simulink model "Scenario_17_v2"  (R2020b)
settings: Solver=ode1  StartTime=0.0  StopTime=10  FixedStep=Ts  MaxStep=Ts  MinStep=Ts/50  RelTol=1e-3
values from neighbouring files (symbols this model uses):
  c0 = c0_zeb    (= 6.57988e-09)    [Scenario_17_parameters_v2.m]    (also in Scenario_1_parameters_v2.m; Scenario_2_parameters_v2.m; Scenario_3_parameters_v2.m)
  c1 = c1_zeb    (= 9.15905e-09)    [Scenario_17_parameters_v2.m]    (also in Scenario_1_parameters_v2.m; Scenario_2_parameters_v2.m; Scenario_3_parameters_v2.m)
  fg = 50    [Scenario_17_parameters_v2.m]    (also in Scenario_1_parameters_v2.m; Scenario_2_parameters_v2.m; Scenario_3_parameters_v2.m)
  G11gen = 0.50    (= 0.5)    [Scenario_17_parameters_v2.m]
  G1gen = 0.4692    [Scenario_17_parameters_v2.m]    (also in Scenario_1_parameters_v2.m = 0.1; Scenario_2_parameters_v2.m = 0.298581; Scenario_3_parameters_v2.m = 0.65)
  G5gen = 0.75    [Scenario_17_parameters_v2.m]    (also in Scenario_1_parameters_v2.m = 0.8; Scenario_2_parameters_v2.m = 0.8; Scenario_3_parameters_v2.m = 0.705)
  G6gen = 0.90    (= 0.9)    [Scenario_17_parameters_v2.m]    (also in Scenario_1_parameters_v2.m; Scenario_2_parameters_v2.m = 0.81797; Scenario_3_parameters_v2.m = 0.45)
  G7gen = 0.20    (= 0.2)    [Scenario_17_parameters_v2.m]    (also in Scenario_1_parameters_v2.m = 0.5227; Scenario_2_parameters_v2.m = 0.5098; Scenario_3_parameters_v2.m = 0.4)
  G8gen = 0.58    [Scenario_17_parameters_v2.m]    (also in Scenario_3_parameters_v2.m = 0.65)
  G9gen = 0.8833    [Scenario_17_parameters_v2.m]    (also in Scenario_3_parameters_v2.m = 0.9)
  Iovc = 1.2    [Scenario_17_parameters_v2.m]    (also in Scenario_1_parameters_v2.m; Scenario_2_parameters_v2.m; Scenario_3_parameters_v2.m)
  l0 = l0_zeb    (= 0.00368)    [Scenario_17_parameters_v2.m]    (also in Scenario_1_parameters_v2.m; Scenario_2_parameters_v2.m; Scenario_3_parameters_v2.m)
  l1 = l1_zeb    (= 0.00128)    [Scenario_17_parameters_v2.m]    (also in Scenario_1_parameters_v2.m; Scenario_2_parameters_v2.m; Scenario_3_parameters_v2.m)
  L11dem = 0.02    [Scenario_17_parameters_v2.m]
  L12dem = 0.01    [Scenario_17_parameters_v2.m]    (also in Scenario_3_parameters_v2.m = 0.02)
  L1dem = 0.25    [Scenario_17_parameters_v2.m]    (also in Scenario_3_parameters_v2.m = 0.1)
  L3dem = 0.30    (= 0.3)    [Scenario_17_parameters_v2.m]    (also in Scenario_1_parameters_v2.m = 0.1; Scenario_2_parameters_v2.m = 0.1; Scenario_3_parameters_v2.m = 0.2)
  L5dem = 0.25    [Scenario_17_parameters_v2.m]    (also in Scenario_1_parameters_v2.m = 0.35; Scenario_2_parameters_v2.m = 0.35; Scenario_3_parameters_v2.m = 0.1)
  L9dem = 0.15    [Scenario_17_parameters_v2.m]    (also in Scenario_3_parameters_v2.m = 0.1)
  Pr = Sr*PF    (= 1600500000)    [Scenario_17_parameters_v2.m]    (also in Scenario_1_parameters_v2.m = 1472500000; Scenario_2_parameters_v2.m = 1805000000; Scenario_3_parameters_v2.m = 12740000000)
  Qr = sqrt(Sr^2 - Pr^2)    [Scenario_17_parameters_v2.m]    (also in Scenario_1_parameters_v2.m; Scenario_2_parameters_v2.m; Scenario_3_parameters_v2.m)
  r0 = r0_zeb    (= 0.39362)    [Scenario_17_parameters_v2.m]    (also in Scenario_1_parameters_v2.m; Scenario_2_parameters_v2.m; Scenario_3_parameters_v2.m)
  r1 = r1_zeb    (= 0.06862)    [Scenario_17_parameters_v2.m]    (also in Scenario_1_parameters_v2.m; Scenario_2_parameters_v2.m; Scenario_3_parameters_v2.m)
  Rtpu = Xtpu/40    (= 0.0025)    [Scenario_17_parameters_v2.m]    (also in Scenario_1_parameters_v2.m = 0.00375; Scenario_2_parameters_v2.m = 0.00375; Scenario_3_parameters_v2.m)
  S11non = 50e6    (= 50000000)    [Scenario_17_parameters_v2.m]
  S1non = 700e6    (= 700000000)    [Scenario_17_parameters_v2.m]    (also in Scenario_1_parameters_v2.m = 400000000; Scenario_2_parameters_v2.m = 400000000; Scenario_3_parameters_v2.m = 1000000000)
  S5non = 400e6    (= 400000000)    [Scenario_17_parameters_v2.m]    (also in Scenario_1_parameters_v2.m = 500000000; Scenario_2_parameters_v2.m = 500000000; Scenario_3_parameters_v2.m = 2000000000)
  S6non = 150e6    (= 150000000)    [Scenario_17_parameters_v2.m]    (also in Scenario_1_parameters_v2.m = 400000000; Scenario_2_parameters_v2.m = 400000000; Scenario_3_parameters_v2.m = 3000000000)
  S7non = 1500e6    (= 1500000000)    [Scenario_17_parameters_v2.m]    (also in Scenario_1_parameters_v2.m = 200000000; Scenario_2_parameters_v2.m = 200000000; Scenario_3_parameters_v2.m = 4000000000)
  S8non = 600e6    (= 600000000)    [Scenario_17_parameters_v2.m]    (also in Scenario_3_parameters_v2.m = 2000000000)
  S9non = 200e6    (= 200000000)    [Scenario_17_parameters_v2.m]    (also in Scenario_3_parameters_v2.m = 1500000000)
  tonvsc = 0    [Scenario_17_parameters_v2.m]    (also in Scenario_1_parameters_v2.m; Scenario_2_parameters_v2.m; Scenario_3_parameters_v2.m = 0.0001)
  Ts = 50e-6    (= 5e-05)    [Scenario_17_parameters_v2.m]    (also in Scenario_1_parameters_v2.m = 0.0002; Scenario_2_parameters_v2.m = 2e-05; Scenario_3_parameters_v2.m = 0.0001)
  Vhv = 220e3    (= 220000)    [Scenario_17_parameters_v2.m]    (also in Scenario_1_parameters_v2.m; Scenario_2_parameters_v2.m; Scenario_3_parameters_v2.m)
  Vmv = 22e3    (= 22000)    [Scenario_17_parameters_v2.m]    (also in Scenario_1_parameters_v2.m; Scenario_2_parameters_v2.m; Scenario_3_parameters_v2.m)
  w_pll = 2*pi*80    (= 502.654824574)    [Scenario_17_parameters_v2.m]    (also in Scenario_1_parameters_v2.m; Scenario_2_parameters_v2.m; Scenario_3_parameters_v2.m)
  wc1 = wsw1/10    (= 848.230016469)    [Scenario_17_parameters_v2.m]    (also in Scenario_1_parameters_v2.m; Scenario_2_parameters_v2.m; Scenario_3_parameters_v2.m)
  wdc1 = wc1/10    (= 84.8230016469)    [Scenario_17_parameters_v2.m]    (also in Scenario_1_parameters_v2.m; Scenario_2_parameters_v2.m; Scenario_3_parameters_v2.m)
  wpq1 = wc1/10    (= 84.8230016469)    [Scenario_17_parameters_v2.m]    (also in Scenario_1_parameters_v2.m; Scenario_2_parameters_v2.m; Scenario_3_parameters_v2.m)
  wsw1 = ksw1*2*pi*fg    (= 8482.30016469)    [Scenario_17_parameters_v2.m]    (also in Scenario_1_parameters_v2.m; Scenario_2_parameters_v2.m; Scenario_3_parameters_v2.m)
  Xtpu = 0.10    (= 0.1)    [Scenario_17_parameters_v2.m]    (also in Scenario_1_parameters_v2.m = 0.15; Scenario_2_parameters_v2.m = 0.15; Scenario_3_parameters_v2.m)
undefined symbols (not defined in the file or in its folder): D11, Delta, Newton, Raphson
libraries: powerlib x349, simulink_extras x215, powerlib_meascontrol x165, pid_lib x81, simulink x48, eeTransforms x42, spsFirstOrderFilterLib x28, eePwmGeneratorTwoLevel x7
(part 2 of 31)

== system Scenario_17_v2/B7 ==
  Current Measurement : powerlib/Measurements/Current Measurement  PhasorSimulation=off  OutputType=Complex  PSBequivalent=0
  Current Measurement1 : powerlib/Measurements/Current Measurement  PhasorSimulation=off  OutputType=Complex  PSBequivalent=0
  Current Measurement2 : powerlib/Measurements/Current Measurement  PhasorSimulation=off  OutputType=Complex  PSBequivalent=0
  Gain : Gain
  Gain1 : Gain
  Ground : powerlib/Elements/Ground  LConnTagsString=a
  Ground1 : powerlib/Elements/Ground  LConnTagsString=a
  Ground2 : powerlib/Elements/Ground  LConnTagsString=a
  Load Flow Bus : powerlib/Measurements/Load Flow Bus  LConnTagsString=a  Phases=single  Connectors=on one side  ID=BUS7  Vbase=Vhv  Vref=1  Vangle=0  VLF=1  VLFb=1  VLFc=1  angleLF=0  angleLFb=0  angleLFc=0
  Mux : Mux  Inputs=3
  Mux1 : Mux  Inputs=3
  Voltage Measurement : powerlib/Measurements/Voltage Measurement  PhasorSimulation=off  OutputType=Complex  PSBequivalent=0
  Voltage Measurement1 : powerlib/Measurements/Voltage Measurement  PhasorSimulation=off  OutputType=Complex  PSBequivalent=0
  Voltage Measurement2 : powerlib/Measurements/Voltage Measurement  PhasorSimulation=off  OutputType=Complex  PSBequivalent=0
  A : PMIOPort  Side=Left
  B : PMIOPort  Port=2  Side=Left
  C : PMIOPort  Port=3  Side=Left
  a : PMIOPort  Port=4  Side=Right
  b : PMIOPort  Port=5  Side=Right
  c : PMIOPort  Port=6  Side=Right
  tag scope: I7=global, V7=global
  wires:
  Voltage Measurement2/1 -> Mux/3
  Voltage Measurement1/1 -> Mux/2
  Voltage Measurement/1 -> Mux/1
  Current Measurement/1 -> Mux1/1
  Current Measurement1/1 -> Mux1/2
  Current Measurement2/1 -> Mux1/3
  Mux/1 -> Gain/1
  Gain/1 -> [V7]
  Mux1/1 -> Gain1/1
  Gain1/1 -> [I7]
  connections:
  Current Measurement/RConn1 -- a/RConn1
  Current Measurement1/LConn1 -- Voltage Measurement1/LConn1 -- B/RConn1
  Current Measurement2/LConn1 -- Voltage Measurement2/LConn1 -- C/RConn1
  Current Measurement/LConn1 -- Voltage Measurement/LConn1 -- Load Flow Bus/LConn1 -- A/RConn1
  Current Measurement1/RConn1 -- b/RConn1
  Current Measurement2/RConn1 -- c/RConn1
  Ground/LConn1 -- Voltage Measurement/LConn2
  Ground1/LConn1 -- Voltage Measurement1/LConn2
  Ground2/LConn1 -- Voltage Measurement2/LConn2

== system Scenario_17_v2/B8 ==
  Current Measurement : powerlib/Measurements/Current Measurement  PhasorSimulation=off  OutputType=Complex  PSBequivalent=0
  Current Measurement1 : powerlib/Measurements/Current Measurement  PhasorSimulation=off  OutputType=Complex  PSBequivalent=0
  Current Measurement2 : powerlib/Measurements/Current Measurement  PhasorSimulation=off  OutputType=Complex  PSBequivalent=0
  Gain : Gain
  Gain1 : Gain
  Ground : powerlib/Elements/Ground  LConnTagsString=a
  Ground1 : powerlib/Elements/Ground  LConnTagsString=a
  Ground2 : powerlib/Elements/Ground  LConnTagsString=a
  Load Flow Bus : powerlib/Measurements/Load Flow Bus  LConnTagsString=a  Phases=single  Connectors=on one side  ID=BUS8  Vbase=Vhv  Vref=1  Vangle=0  VLF=1  VLFb=1  VLFc=1  angleLF=0  angleLFb=0  angleLFc=0
  Mux : Mux  Inputs=3
  Mux1 : Mux  Inputs=3
  Voltage Measurement : powerlib/Measurements/Voltage Measurement  PhasorSimulation=off  OutputType=Complex  PSBequivalent=0
  Voltage Measurement1 : powerlib/Measurements/Voltage Measurement  PhasorSimulation=off  OutputType=Complex  PSBequivalent=0
  Voltage Measurement2 : powerlib/Measurements/Voltage Measurement  PhasorSimulation=off  OutputType=Complex  PSBequivalent=0
  A : PMIOPort  Side=Left
  B : PMIOPort  Port=2  Side=Left
  C : PMIOPort  Port=3  Side=Left
  a : PMIOPort  Port=4  Side=Right
  b : PMIOPort  Port=5  Side=Right
  c : PMIOPort  Port=6  Side=Right
  tag scope: I8=global, V8=global
  wires:
  Voltage Measurement2/1 -> Mux/3
  Voltage Measurement1/1 -> Mux/2
  Voltage Measurement/1 -> Mux/1
  Current Measurement/1 -> Mux1/1
  Current Measurement1/1 -> Mux1/2
  Current Measurement2/1 -> Mux1/3
  Mux/1 -> Gain/1
  Gain/1 -> [V8]
  Mux1/1 -> Gain1/1
  Gain1/1 -> [I8]
  connections:
  Current Measurement/RConn1 -- a/RConn1
  Current Measurement1/LConn1 -- Voltage Measurement1/LConn1 -- B/RConn1
  Current Measurement2/LConn1 -- Voltage Measurement2/LConn1 -- C/RConn1
  Current Measurement/LConn1 -- Voltage Measurement/LConn1 -- Load Flow Bus/LConn1 -- A/RConn1
  Current Measurement1/RConn1 -- b/RConn1
  Current Measurement2/RConn1 -- c/RConn1
  Ground/LConn1 -- Voltage Measurement/LConn2
  Ground1/LConn1 -- Voltage Measurement1/LConn2
  Ground2/LConn1 -- Voltage Measurement2/LConn2

== system Scenario_17_v2/B9 ==
  Current Measurement : powerlib/Measurements/Current Measurement  PhasorSimulation=off  OutputType=Complex  PSBequivalent=0
  Current Measurement1 : powerlib/Measurements/Current Measurement  PhasorSimulation=off  OutputType=Complex  PSBequivalent=0
  Current Measurement2 : powerlib/Measurements/Current Measurement  PhasorSimulation=off  OutputType=Complex  PSBequivalent=0
  Gain : Gain
  Gain1 : Gain
  Ground : powerlib/Elements/Ground  LConnTagsString=a
  Ground1 : powerlib/Elements/Ground  LConnTagsString=a
  Ground2 : powerlib/Elements/Ground  LConnTagsString=a
  Load Flow Bus : powerlib/Measurements/Load Flow Bus  LConnTagsString=a  Phases=single  Connectors=on one side  ID=BUS9  Vbase=Vmv  Vref=1  Vangle=0  VLF=1  VLFb=1  VLFc=1  angleLF=-33.63  angleLFb=0  angleLFc=0
  Mux : Mux  Inputs=3
  Mux1 : Mux  Inputs=3
  Voltage Measurement : powerlib/Measurements/Voltage Measurement  PhasorSimulation=off  OutputType=Complex  PSBequivalent=0
  Voltage Measurement1 : powerlib/Measurements/Voltage Measurement  PhasorSimulation=off  OutputType=Complex  PSBequivalent=0
  Voltage Measurement2 : powerlib/Measurements/Voltage Measurement  PhasorSimulation=off  OutputType=Complex  PSBequivalent=0
  A : PMIOPort  Side=Left
  B : PMIOPort  Port=2  Side=Left
  C : PMIOPort  Port=3  Side=Left
  a : PMIOPort  Port=4  Side=Right
  b : PMIOPort  Port=5  Side=Right
  c : PMIOPort  Port=6  Side=Right
  tag scope: I9=global, V9=global
  wires:
  Voltage Measurement2/1 -> Mux/3
  Voltage Measurement1/1 -> Mux/2
  Voltage Measurement/1 -> Mux/1
  Current Measurement/1 -> Mux1/1
  Current Measurement1/1 -> Mux1/2
  Current Measurement2/1 -> Mux1/3
  Mux/1 -> Gain/1
  Gain/1 -> [V9]
  Mux1/1 -> Gain1/1
  Gain1/1 -> [I9]
  connections:
  Current Measurement/RConn1 -- a/RConn1
  Current Measurement1/LConn1 -- Voltage Measurement1/LConn1 -- B/RConn1
  Current Measurement2/LConn1 -- Voltage Measurement2/LConn1 -- C/RConn1
  Current Measurement/LConn1 -- Voltage Measurement/LConn1 -- Load Flow Bus/LConn1 -- A/RConn1
  Current Measurement1/RConn1 -- b/RConn1
  Current Measurement2/RConn1 -- c/RConn1
  Ground/LConn1 -- Voltage Measurement/LConn2
  Ground1/LConn1 -- Voltage Measurement1/LConn2
  Ground2/LConn1 -- Voltage Measurement2/LConn2

== system Scenario_17_v2/G1 ==
  note: Synchronous Machine Model according to ENTSO-E
  note: Nomenclature (according to IEEE Std 421.1-2007):
      | Efd = Exciter output voltage (generator field voltage)
      | Ifd = Exciter output current (generator field current)
      | Vf = Excitation system stabilizer signal
      | Vfe = Signal proportional to exciter field current
      | Vl = Limiters and protective elements feedback
      | Vr = Regulator output
      | Vs = Power System Stabilizer (PSS) output
      | Vsi = Power System Stabilizer (PSS) inputs (shaft speed, frequency, generator electric power, and others
      | Vt = Generator terminal voltage
      | It = Generator terminal current
      | Vref = Voltage regulator reference signal
      | Vc = terminal voltage transducer output
  Bus Selector : BusSelector  OutputSignals=dw,w,vq,vd,iq,id,Peo,Te,delta,dtheta,ias,ibs,ics
  Constant : Constant  Value=G1gen
  Exciter System : Subsystem
  Real-Imag to Complex : RealImagToComplex
  Real-Imag to Complex1 : RealImagToComplex
  Ref voltage (p.u) : Constant  Value=1.00
  Snubber : powerlib/Elements/Three-Phase Parallel RLC Load  LConnTagsString=A|B|C  Configuration=Y (grounded)  NominalVoltage=Vmv  Vabc=[1e3 1e3 1e3]  Vabcp=[1e3 1e3 1e3]  NominalFrequency=fg  UnbalancedPower=off  ActivePower=S1non*0.03  InductivePower=0  CapacitivePower=0  Pabc=[10e3 9e3 11e3]  QLabc=[100 90 110]  QCabc=[100 90 110]  Pabcp=[10e3 9e3 11e3]  QLabcp=[100 90 110]  QCabcp=[100 90 110]  Measurements=None  LoadType=constant Z
  Speed Governor : Subsystem  mask{R=0.05, T1=0.5, T2=3, T3=10, Dt=0, Vmin=0, Vmax=10, P0=G1gen}
      mask prompts: R "Controller droop (R)"; T1 "Governor time constant (T1)(sec)"; T2 "Turbine derivative time constant (T2)(sec)"; T3 "Turbine delay time constant (T3)(sec)"; Dt "Frictional losses factor (Dt)"; Vmin "Minimum gate limit (Vmin)(p.u)"; Vmax "Maximum gate limit (Vmax)(p.u)"; P0 "Initial power (p.u)"
      mask Display:
      | disp('TGOV')
      | 
      | port_label('input',1,'Pref')
      | port_label('input',2,'dw')
      | 
      | port_label('output',1,'Pm')
  Synchronous Machine pu Standard : powerlib/Machines/Synchronous Machine pu Standard  Commented=on  PresetModel=No  MechanicalLoad=Mechanical power Pm  ShowDetailedParameters=on  RotorType=Salient-pole  Units=per unit standard parameters  MeasurementBus=on  NominalParameters=[S1non Vmv fg]  Reactances1=[ 1.81, 0.3, 0.23, 1.76, 0.65, 0.25, 0.15 ]  Reactances2=[1.25 0.333 0.292 1.0 0.292 0.15]  dAxisTimeConstants=Open-circuit  qAxisTimeConstants=Open-circuit  TimeConstants1="[6.6  0.05  0.10]"  TimeConstants2=[ 8.0, 0.03, 1.0, 0.07 ]  TimeConstants3="[  4.49  0.0681  0.0513  ]"  TimeConstants4=[ 8.0, 0.03, 0.3371, 0.0295 ]  TimeConstants5=[ 1.01, 0.053, 0.1 ]  TimeConstants6=[ 1.3201, 0.023, 1.0, 0.07 ]  TimeConstants7=[0.012 0.003 0.003]  TimeConstants8=[ 1.3201, 0.0231, 0.3371, 0.0295 ]  StatorResistance=0.01  Mechanical=[6 0 2]  PolePairs=20  InitialConditions=[0 -75.6448 0.296556 0.296556 0.296556 -18.3521 -138.352 101.648 1.17158]  SetSaturation=off  Saturation=[0.6404,0.7127,0.8441,0.9214,0.9956,1.082,1.19,1.316,1.457;0.7,0.7698,0.8872,0.9466,0.9969,1.046,1.1,1.151,1.201]  LoadFlowParameters=[2 200000000 0 0 0]  TsPowergui=0  TsBlock=-1  IterativeModel=Trapezoidal non iterative  IterativeDiscreteModel=Trapezoidal non iterative  BusType=swing  Pref=0  Qref=0  Qmin=-inf  Qmax=inf  PLF=0  QLF=0
  Synchronous Machine pu Standard1 : powerlib/Machines/Synchronous Machine pu Standard  PresetModel=No  MechanicalLoad=Mechanical power Pm  ShowDetailedParameters=on  RotorType=Salient-pole  Units=per unit standard parameters  MeasurementBus=on  NominalParameters=[S1non Vmv fg]  Reactances1=[ 1.81, 0.3, 0.23, 1.76, 0.65, 0.25, 0.15 ]  Reactances2=[1.25 0.333 0.292 1.0 0.292 0.15]  dAxisTimeConstants=Open-circuit  qAxisTimeConstants=Open-circuit  TimeConstants1="[5  0.002  0.002]"  TimeConstants2=[ 8.0, 0.03, 1.0, 0.07 ]  TimeConstants3="[  4.49  0.0681  0.0513  ]"  TimeConstants4=[ 8.0, 0.03, 0.3371, 0.0295 ]  TimeConstants5=[ 1.01, 0.053, 0.1 ]  TimeConstants6=[ 1.3201, 0.023, 1.0, 0.07 ]  TimeConstants7=[0.012 0.003 0.003]  TimeConstants8=[ 1.3201, 0.0231, 0.3371, 0.0295 ]  StatorResistance=0.01  Mechanical=[6 0 2]  PolePairs=20  InitialConditions=[0 -66.5325 0.472095 0.472095 0.472095 -8.44863 -128.449 111.551 1.23328]  SetSaturation=off  Saturation=[0.6404,0.7127,0.8441,0.9214,0.9956,1.082,1.19,1.316,1.457;0.7,0.7698,0.8872,0.9466,0.9969,1.046,1.1,1.151,1.201]  LoadFlowParameters=[2 200000000 0 0 0]  TsPowergui=0  TsBlock=-1  IterativeModel=Trapezoidal non iterative  IterativeDiscreteModel=Trapezoidal non iterative  BusType=swing  Pref=G1gen*S1non  Qref=0.1357*S1non  Qmin=-inf  Qmax=inf  PLF=0  QLF=0
  Three-Phase Transformer (Two Windings) : powerlib/Elements/Three-Phase Transformer (Two Windings)  Winding1Connection=Delta (D11)  Winding2Connection=Yg  CoreType=Three single-phase transformers  SetSaturation=off  Hysteresis=off  DataFile='hysteresis'  SetInitialFlux=off  Measurements=None  UNITS=pu  NominalPower=[S1non , fg ]  Winding1=[Vmv 0.00125 0.05]  Winding2=[Vhv 0.00125 0.05]  Rm=5000  Lm=5000  L0=0.5  Saturation=[ 0,0 ; 0.0024,1.2 ; 1.0,1.52 ]  InitialFluxes=[ 0.8 , -0.8 , 0.7 ]  BreakLoop=off  DiscreteSolver=Trapezoidal iterative  DataType=off  TransfoNumber=1
  A : PMIOPort  Side=Right
  B : PMIOPort  Port=2  Side=Right
  C : PMIOPort  Port=3  Side=Right
  tag scope: Te1=global, wm1=global
  wires:
  Bus Selector/1 -> Speed Governor/2(dw), Exciter System/1(<dw>)  "<dw>"
  Bus Selector/4 -> Real-Imag to Complex/2  "<vd>"
  Bus Selector/3 -> Real-Imag to Complex/1  "<vq>"
  Bus Selector/5 -> Real-Imag to Complex1/1  "<iq>"
  Bus Selector/6 -> Real-Imag to Complex1/2  "<id>"
  Real-Imag to Complex/1 -> Exciter System/3(Vt)
  Real-Imag to Complex1/1 -> Exciter System/4(It)
  Bus Selector/8 -> [Te1]  "<Te>"
  Speed Governor/1(Pm) -> Synchronous Machine pu Standard1/1
  Exciter System/1(Efd) -> Synchronous Machine pu Standard1/2
  Synchronous Machine pu Standard1/1 -> Bus Selector/1
  Constant/1 -> Speed Governor/1(RefL)
  Bus Selector/2 -> [wm1]  "<w>"
  Bus Selector/7 -> Exciter System/5(<Peo>)  "<Peo>"
  Ref voltage (p.u)/1 -> Exciter System/2(Vref)
  Bus Selector/9 -> ?  "<delta>"
  Bus Selector/10 -> ?  "<dtheta>"
  Bus Selector/11 -> ?  "<ias>"
  Bus Selector/12 -> ?  "<ibs>"
  Bus Selector/13 -> ?  "<ics>"
  connections:
  Three-Phase Transformer (Two Windings)/LConn1 -- Synchronous Machine pu Standard1/RConn1 -- Snubber/LConn1
  Three-Phase Transformer (Two Windings)/LConn3 -- Synchronous Machine pu Standard1/RConn3 -- Snubber/LConn3
  Three-Phase Transformer (Two Windings)/LConn2 -- Synchronous Machine pu Standard1/RConn2 -- Snubber/LConn2
  Three-Phase Transformer (Two Windings)/RConn1 -- A/RConn1
  Three-Phase Transformer (Two Windings)/RConn2 -- B/RConn1
  Three-Phase Transformer (Two Windings)/RConn3 -- C/RConn1

== system Scenario_17_v2/G11new ==
  Bus Selector : BusSelector  OutputSignals=Pabc,Qabc,f
  Constant : Constant  Value=S11non*G11gen
  Constant1 : Constant  Value=20e6
  VSC v2 : Subsystem  mask{vscmod=EMT Average, fg=fg, Vhv=Vmv, Vmv=Vmv, Pconv=S11non, Rtpu=Rtpu, Xtpu=Xtpu, qmode=Active power, dmode=Reactive power, wsw=wsw1, wn_pll=w_pll, wc=wc1, wpq=wpq1, wdc=wdc1, koc=Iovc, Cdc=3100e-6, tfilt=1*(1/wsw1), negseq_en=off, fdroop_en=off, Vacdroop_en=off, LVRT_en=off, Kfdroop=0.05, fdroop_per=10, Kvdroop=0.1, Vacdroop_per=10, Vlvrt0=0.9, Vlvrt_min=0.5, Qmax_lvrt=0.9, V0pu=1.1206, theta0=-44.38, P0=S11non*G11gen, Q0=20e6}
      mask prompts: vscmod "VSC Model"; fg "AC grid frequency (Hz)"; Vhv "Grid-side voltage (V)(LL-rms)"; Vmv "Converter-side voltage (V)(LL-rms)"; Pconv "Converter nominal power (VA)"; Rtpu "Resistance seen by the converter (p.u)"; Xtpu "Reactance seen by the converter (p.u)"; qmode "q-axis control mode"; dmode "d-axis control mode"; wsw "Switching frequency (rad/s)"; wn_pll "PLL filter natural frequency"; wc "Current-control bandwidth (rad/s)"; wpq "PQ control bandwidth (rad/s)"; wdc "DC Voltage control bandwidth(rad/s)"; koc "Overcurrent factor (p.u)"; Cdc "DC-side total capacitance (F)"; tfilt "Vabc filter time constant (s)"; negseq_en "Enable negative sequence control"; fdroop_en "Enable frequency droop"; Vacdroop_en "Enable AC voltage droop"; LVRT_en "Enable LVRT"; Kfdroop "Frequency droop (p.u)"; fdroop_per "Percentage of converter power to contribute with droop (%)"; Kvdroop "Voltage droop (p.u)"; Vacdroop_per "Percentage of converter power to contribute with droop (%)"; Vlvrt0 "initial voltage (p.u)"; Vlvrt_min "minimum voltage (p.u)"; Qmax_lvrt "max power injected at min voltage (p.u)"; V0pu "Initial terminal voltage magnitude (pu)"; theta0 "Initial terminal voltage angle (deg)"; P0 "Initial active power (W)"; Q0 "Initial reactive power (VAr)"
      mask init:
      | %% ----------------------VSC Parameters-------------------------- %%
      | j = 1i;
      | r = Vhv/Vmv;                    % Transformer ratio
      | Vmvpk = Vmv*sqrt(2)/sqrt(3);    % Converter-side voltage phase-to-ground peak-to-peak
      | Vhvpk = Vhv*sqrt(2)/sqrt(3);    % Grid-side voltage phase-to-ground peak-to-peak  
      | Vdc = 2*Vhvpk;                  % Nominal DC voltage 
      | ksw = round(wsw/(2*pi*fg));      % Calculates switching ratio
      | Iconvbase = 2*Pconv/(3*Vmvpk);  % Converter base current (A)
      | Zbmv = Vmv^2/Pconv;             % Base voltage referred to the converter side
      | Imax = koc*Iconvbase;   % Converter maximum output current
      | %Cdc = 2*Hvsc*Pconv/Vdc^2;       % DC capacitor
      | 
      | Xt = Xtpu*Zbmv;        % p.u to (Ohms)
      | Lt = Xt/(2*pi*fg);              % p.u to (H)
      | Rt = Rtpu*Zbmv;        % p.u. to (Ohms)
      | 
      | % -------------LVRT--------------%
      | Klvrt = Qmax_lvrt/(Vlvrt_min-Vlvrt0); % Defines LVRT inclination of the V/I LVRT characteristic
      | 
      | % ------------ PLL ------------- %
      | zeta_pll = 1/sqrt(2);           % Damping
      | kp_pll = 2*zeta_pll*wn_pll/(Vmvpk);
      | tau_pll = 2*zeta_pll/wn_pll;
      | 
      | % ------------ Inner-loop (current control) ------------ %
      | kp_c = Lt*wc; 
      | ti_c = Lt/Rt;
      | 
      | % -------- Outer-loop (voltage and/or power control)
      | % --- PQ closed-loop control ----
      | ti_pq = 1/wc;
      | kp_pq = 2/3*ti_pq*wpq*1/Vmvpk;
      | 
      | % --- Vdc control ----
      | damp_dc = 1/sqrt(2);
      | kp_dc = 2*Cdc*damp_dc*wdc; 
      | ki_dc = Cdc*wdc^2;
      | 
      | %% ---------------------Mask operations----------------------------%%
      | 
      | % If the box is unchecked, we set the bias value to zero
      | if ~fdroop_en; end
      | if ~Vacdroop_en; end
      | if ~LVRT_en; Klvrt = 0;  end
      | 
      | %% -------------------- Variant Subsystem ----------------------- %%
      | choice = get_param(gcb,'vscmod'); % Get choice from list
      | VSS_model = [gcb, '/VSC Model'];  % VSC electrical Model
      | VSS_meas = [gcb, '/VSC Control/Measurements']; % Measurements (PLL, Park transformation, etc)
      | VSS_mod = [gcb, '/VSC Control/Modulation']; % Modulation or reference voltage/current generation
      | VSS_ctr = [gcb, '/VSC Control/Control loops']; % Modulation or reference voltage/current generation
      | 
      | 
      | if strcmp(choice,'EMT Switching')
      |     set_param(VSS_model, 'LabelModeActiveChoice', 'EMT_SW');
      |     set_param(VSS_meas, 'LabelModeActiveChoice', 'EMT');
      |     set_param(VSS_mod, 'LabelModeActiveChoice', 'EMT_SW');
      |     set_param(VSS_ctr, 'LabelModeActiveChoice', 'EMT_and_QEMT');
      |     
      | elseif strcmp(choice,'EMT Average')
      |     set_param(VSS_model, 'LabelModeActiveChoice', 'EMT_AVG');
      |     set_param(VSS_meas, 'LabelModeActiveChoice', 'EMT');
      |     set_param(VSS_mod, 'LabelModeActiveChoice', 'EMT_AVG');
      |     set_param(VSS_ctr, 'LabelModeActiveChoice', 'EMT_and_QEMT');
      |     %set_param([VSS_meas '/EMT/Vabc filter'],'Commented','through')
      |     tfilt = 0; % No filtering in Average model
      |     
      | elseif strcmp(choice,'Phasor Quasi-EMT')
      |     set_param(VSS_model, 'LabelModeActiveChoice', 'Phasor');
      |     set_param(VSS_meas, 'LabelModeActiveChoice', 'Phasor');
      |     set_param(VSS_mod, 'LabelModeActiveChoice', 'Phasor_QEMT');
      |     set_param(VSS_ctr, 'LabelModeActiveChoice', 'EMT_and_QEMT');
      |     
      | elseif strcmp(choice,'Phasor I-1st')
      |     set_param(VSS_model, 'LabelModeActiveChoice', 'Phasor');
      |     set_param(VSS_meas, 'LabelModeActiveChoice', 'Phasor');
      |     set_param(VSS_mod, 'LabelModeActiveChoice', 'Phasor_I_and_PQ');
      |     set_param(VSS_ctr, 'LabelModeActiveChoice', 'Phasor_I_1st');
      |     
      | elseif strcmp(choice,'Phasor I-ref')
      |     set_param(VSS_model, 'LabelModeActiveChoice', 'Phasor');
      | 	set_param(VSS_meas, 'LabelModeActiveChoice', 'Phasor');
      |     set_param(VSS_mod, 'LabelModeActiveChoice', 'Phasor_I_and_PQ');
      |     set_param(VSS_ctr, 'LabelModeActiveChoice', 'Phasor_I_ref');
      |     
      | elseif strcmp(choice,'Phasor PQ-1st')
      |     set_param(VSS_model, 'LabelModeActiveChoice', 'Phasor');
      |     set_param(VSS_meas, 'LabelModeActiveChoice', 'Phasor');
      |     set_param(VSS_mod, 'LabelModeActiveChoice', 'Phasor_I_and_PQ');
      |     set_param(VSS_ctr, 'LabelModeActiveChoice', 'Phasor_PQ');
      | end
      | 
      | 
      | %% ------------------------- Converter initialization -----------------------------
      | 
      | %-------------- Electrical part ----------------------
      | theta0 = theta0*pi/180; % deg to rad
      | 
      | Vgmag = V0pu*Vhv/sqrt(3); % Phase Voltage magnitude (LG,RMS)
      | Xt = Xtpu*Zbmv; % Converting the reactance the converter sees to Ohms
      | 
      | % Grid voltage in rectangular format, with reference to the MV-side (divided by the transformer relation)
      | [Vgr,Vgi] = pol2cart(theta0,Vgmag/r);
      | Vg = complex(Vgr,Vgi);
      | 
      | % Complex power
      | S0 = complex(P0,Q0);
      | 
      | % Converter output current (RMS), with reference to the MV side
      | Ic = conj(S0/(3*Vg));
      | 
      | % Converter internal voltage (LG,RMS), with reference to the MV side
      | Vc = Vg + Ic*(Rt + j*Xt);
      | 
      | %------------------- Converter part ----------------
      | 
      | % ---------- PLL -----------
      | % The angle used in dq transformation is different in EMT and in Phasor
      | if (strcmp(choice,'EMT Switching') || strcmp(choice,'EMT Average'))
      |     thetaPLL = pi + theta0;
      | elseif (strcmp(choice,'Phasor Quasi-EMT') || strcmp(choice,'Phasor I-1st') || strcmp(choice,'Phasor I-ref') || strcmp(choice,'Phasor PQ-1st'))
      |     thetaPLL = pi;
      | end
      | 
      | 
      | % ------ dq variables --------
      | 
      | Vgq = imag(Vg*sqrt(2)*exp(-j*(thetaPLL + pi/2))); 
      | Vgd = real(Vg*sqrt(2)*exp(-j*(thetaPLL + pi/2))); 
      | 
      | Vcq = imag(Vc*sqrt(2)*exp(-j*(thetaPLL + pi/2))); 
      | Vcd = real(Vc*sqrt(2)*exp(-j*(thetaPLL + pi/2))); 
      | 
      | Icq = imag(Ic*sqrt(2)*exp(-j*(thetaPLL + pi/2))); 
      | Icd = real(Ic*sqrt(2)*exp(-j*(thetaPLL + pi/2))); 
      | 
      | % ------ Inner loop ------
      | % Now that we know the reference voltage in dq (Vc,qd), the grid voltage in dq (Vg,qd) and the converter
      | % current in dq (Ic,dq), we can calculate the PI controller output in t=0
      | % As we assume zero steady-state error, the proportional part is zero and we calculate only the integrator part (Tc,qd)
      | Tcq = Vcq - Vgq - Xt*Icd;
      | Tcd = Vcd - Vgd + Xt*Icq;
      | 
      | % ------- Outer loop -------
      | % As we know the converter current, and we know that the proportional part is zero, we calculate the
      | % integrator part (To,qd)
      | Toq = Icq;
      | Tod = Icd;
      mask TypeOptions vscmod: EMT Switching | EMT Average | Phasor Quasi-EMT | Phasor I-1st | Phasor I-ref | Phasor PQ-1st
      mask Callback vscmod:
      | % Control parameter visiblity
      | 
      | % Get the value of the Enable Bias checkbox
      | % unchecked = 'off'
      | % checked = 'on'
      | 
      | maskObj = Simulink.Mask.get(gcb);
      | 
      | wn_pll = 'on';
      | wsw = 'on';
      | DC_en = 'off';
      | 
      | vscmod = get_param(gcb,'vscmod');
      |     if strcmp(vscmod,'EMT Switching')
      |       wn_pll = 'on';
      |       wsw = 'on';
      |       tfilt = 'on';
      |     elseif strcmp(vscmod,'EMT Average')
      |         wn_pll = 'on';
      |         wsw = 'off';
      |         tfilt = 'off';
      |     elseif strcmp(vscmod,'Phasor Quasi-EMT')
      |         wn_pll = 'off';
      |         wsw = 'off';
      |         tfilt = 'off';
      |     elseif strcmp(vscmod,'Phasor I-1st')
      |         wn_pll = 'off';
      |         wsw = 'off';
      |         tfilt = 'off';
      |     elseif strcmp(vscmod,'Phasor I-ref')
      |         wn_pll = 'off';
      |         wsw = 'off';
      |         tfilt = 'off';
      |     elseif strcmp(vscmod,'Phasor PQ-1st')
      |         wn_pll = 'off';
      |         wsw = 'off';
      |         tfilt = 'off';
      |     end
      | 
      | fdroop_en = get_param(gcb,'fdroop_en');
      | Vacdroop_en = get_param(gcb,'Vacdroop_en');
      | LVRT_en = get_param(gcb,'LVRT_en');
      | negseq_en = get_param(gcb,'negseq_en');
      | qmode_str = get_param(gcb,'qmode');
      | 
      | 
      | if strcmp(qmode_str,'DC voltage')
      |     DC_en = 'on';
      | else
      |     DC_en = 'off';
      | end
      | 
      | % Set the 'MaskVisibilities' property for each parameters
      |     set_param(gcb,'MaskVisibilities',{'on','on','on','on','on','on','on','on','on',wsw,wn_pll,'on','on','on','on',DC_en,tfilt,'on','on','on','on',fdroop_en,fdroop_en,Vacdroop_en,Vacdroop_en,'on','on','on','on','on','on','on'});
      | 
      | % Make LVRT area visible when it is enabled
      | if strcmp(LVRT_en,'on')
      |   maskObj.getDialogControl('Container_LVRT').Visible = 'on';
      | else
      |     maskObj.getDialogControl('Container_LVRT').Visible = 'off';
      | end
      | 
      | % Note that the value of the bias is not handled here.
      | % See the Initialization tab
      mask TypeOptions qmode: Active power | DC voltage
      mask Callback qmode:
      | % Control parameter visiblity
      | 
      | % Get the value of the Enable Bias checkbox
      | % unchecked = 'off'
      | % checked = 'on'
      | 
      | maskObj = Simulink.Mask.get(gcb);
      | 
      | wn_pll = 'on';
      | wsw = 'on';
      | DC_en = 'off';
      | 
      | vscmod = get_param(gcb,'vscmod');
      |     if strcmp(vscmod,'EMT Switching')
      |       wn_pll = 'on';
      |       wsw = 'on';
      |       tfilt = 'on';
      |     elseif strcmp(vscmod,'EMT Average')
      |         wn_pll = 'on';
      |         wsw = 'off';
      |         tfilt = 'off';
      |     elseif strcmp(vscmod,'Phasor Quasi-EMT')
      |         wn_pll = 'off';
      |         wsw = 'off';
      |         tfilt = 'off';
      |     elseif strcmp(vscmod,'Phasor I-1st')
      |         wn_pll = 'off';
      |         wsw = 'off';
      |         tfilt = 'off';
      |     elseif strcmp(vscmod,'Phasor I-ref')
      |         wn_pll = 'off';
      |         wsw = 'off';
      |         tfilt = 'off';
      |     elseif strcmp(vscmod,'Phasor PQ-1st')
      |         wn_pll = 'off';
      |         wsw = 'off';
      |         tfilt = 'off';
      |     end
      | 
      | fdroop_en = get_param(gcb,'fdroop_en');
      | Vacdroop_en = get_param(gcb,'Vacdroop_en');
      | LVRT_en = get_param(gcb,'LVRT_en');
      | negseq_en = get_param(gcb,'negseq_en');
      | qmode_str = get_param(gcb,'qmode');
      | 
      | 
      | if strcmp(qmode_str,'DC voltage')
      |     DC_en = 'on';
      | else
      |     DC_en = 'off';
      | end
      | 
      | % Set the 'MaskVisibilities' property for each parameters
      |     set_param(gcb,'MaskVisibilities',{'on','on','on','on','on','on','on','on','on',wsw,wn_pll,'on','on','on','on',DC_en,tfilt,'on','on','on','on',fdroop_en,fdroop_en,Vacdroop_en,Vacdroop_en,'on','on','on','on','on','on','on'});
      | 
      | % Make LVRT area visible when it is enabled
      | if strcmp(LVRT_en,'on')
      |   maskObj.getDialogControl('Container_LVRT').Visible = 'on';
      | else
      |     maskObj.getDialogControl('Container_LVRT').Visible = 'off';
      | end
      | 
      | % Note that the value of the bias is not handled here.
      | % See the Initialization tab
      mask TypeOptions dmode: Reactive power | AC voltage
      mask Callback fdroop_en:
      | % Control parameter visiblity
      | 
      | % Get the value of the Enable Bias checkbox
      | % unchecked = 'off'
      | % checked = 'on'
      | 
      | maskObj = Simulink.Mask.get(gcb);
      | 
      | wn_pll = 'on';
      | wsw = 'on';
      | DC_en = 'off';
      | 
      | vscmod = get_param(gcb,'vscmod');
      |     if strcmp(vscmod,'EMT Switching')
      |       wn_pll = 'on';
      |       wsw = 'on';
      |       tfilt = 'on';
      |     elseif strcmp(vscmod,'EMT Average')
      |         wn_pll = 'on';
      |         wsw = 'off';
      |         tfilt = 'off';
      |     elseif strcmp(vscmod,'Phasor Quasi-EMT')
      |         wn_pll = 'off';
      |         wsw = 'off';
      |         tfilt = 'off';
      |     elseif strcmp(vscmod,'Phasor I-1st')
      |         wn_pll = 'off';
      |         wsw = 'off';
      |         tfilt = 'off';
      |     elseif strcmp(vscmod,'Phasor I-ref')
      |         wn_pll = 'off';
      |         wsw = 'off';
      |         tfilt = 'off';
      |     elseif strcmp(vscmod,'Phasor PQ-1st')
      |         wn_pll = 'off';
      |         wsw = 'off';
      |         tfilt = 'off';
      |     end
      | 
      | fdroop_en = get_param(gcb,'fdroop_en');
      | Vacdroop_en = get_param(gcb,'Vacdroop_en');
      | LVRT_en = get_param(gcb,'LVRT_en');
      | negseq_en = get_param(gcb,'negseq_en');
      | qmode_str = get_param(gcb,'qmode');
      | 
      | 
      | if strcmp(qmode_str,'DC voltage')
      |     DC_en = 'on';
      | else
      |     DC_en = 'off';
      | end
      | 
      | % Set the 'MaskVisibilities' property for each parameters
      |     set_param(gcb,'MaskVisibilities',{'on','on','on','on','on','on','on','on','on',wsw,wn_pll,'on','on','on','on',DC_en,tfilt,'on','on','on','on',fdroop_en,fdroop_en,Vacdroop_en,Vacdroop_en,'on','on','on','on','on','on','on'});
      | 
      | % Make LVRT area visible when it is enabled
      | if strcmp(LVRT_en,'on')
      |   maskObj.getDialogControl('Container_LVRT').Visible = 'on';
      | else
      |     maskObj.getDialogControl('Container_LVRT').Visible = 'off';
      | end
      | 
      | % Note that the value of the bias is not handled here.
      | % See the Initialization tab
      mask Callback Vacdroop_en:
      | % Control parameter visiblity
      | 
      | % Get the value of the Enable Bias checkbox
      | % unchecked = 'off'
      | % checked = 'on'
      | 
      | maskObj = Simulink.Mask.get(gcb);
      | 
      | wn_pll = 'on';
      | wsw = 'on';
      | DC_en = 'off';
      | 
      | vscmod = get_param(gcb,'vscmod');
      |     if strcmp(vscmod,'EMT Switching')
      |       wn_pll = 'on';
      |       wsw = 'on';
      |       tfilt = 'on';
      |     elseif strcmp(vscmod,'EMT Average')
      |         wn_pll = 'on';
      |         wsw = 'off';
      |         tfilt = 'off';
      |     elseif strcmp(vscmod,'Phasor Quasi-EMT')
      |         wn_pll = 'off';
      |         wsw = 'off';
      |         tfilt = 'off';
      |     elseif strcmp(vscmod,'Phasor I-1st')
      |         wn_pll = 'off';
      |         wsw = 'off';
      |         tfilt = 'off';
      |     elseif strcmp(vscmod,'Phasor I-ref')
      |         wn_pll = 'off';
      |         wsw = 'off';
      |         tfilt = 'off';
      |     elseif strcmp(vscmod,'Phasor PQ-1st')
      |         wn_pll = 'off';
      |         wsw = 'off';
      |         tfilt = 'off';
      |     end
      | 
      | fdroop_en = get_param(gcb,'fdroop_en');
      | Vacdroop_en = get_param(gcb,'Vacdroop_en');
      | LVRT_en = get_param(gcb,'LVRT_en');
      | negseq_en = get_param(gcb,'negseq_en');
      | qmode_str = get_param(gcb,'qmode');
      | 
      | 
      | if strcmp(qmode_str,'DC voltage')
      |     DC_en = 'on';
      | else
      |     DC_en = 'off';
      | end
      | 
      | % Set the 'MaskVisibilities' property for each parameters
      |     set_param(gcb,'MaskVisibilities',{'on','on','on','on','on','on','on','on','on',wsw,wn_pll,'on','on','on','on',DC_en,tfilt,'on','on','on','on',fdroop_en,fdroop_en,Vacdroop_en,Vacdroop_en,'on','on','on','on','on','on','on'});
      | 
      | % Make LVRT area visible when it is enabled
      | if strcmp(LVRT_en,'on')
      |   maskObj.getDialogControl('Container_LVRT').Visible = 'on';
      | else
      |     maskObj.getDialogControl('Container_LVRT').Visible = 'off';
      | end
      | 
      | % Note that the value of the bias is not handled here.
      | % See the Initialization tab
      mask Callback LVRT_en:
      | % Control parameter visiblity
      | 
      | % Get the value of the Enable Bias checkbox
      | % unchecked = 'off'
      | % checked = 'on'
      | 
      | maskObj = Simulink.Mask.get(gcb);
      | 
      | wn_pll = 'on';
      | wsw = 'on';
      | DC_en = 'off';
      | 
      | vscmod = get_param(gcb,'vscmod');
      |     if strcmp(vscmod,'EMT Switching')
      |       wn_pll = 'on';
      |       wsw = 'on';
      |       tfilt = 'on';
      |     elseif strcmp(vscmod,'EMT Average')
      |         wn_pll = 'on';
      |         wsw = 'off';
      |         tfilt = 'off';
      |     elseif strcmp(vscmod,'Phasor Quasi-EMT')
      |         wn_pll = 'off';
      |         wsw = 'off';
      |         tfilt = 'off';
      |     elseif strcmp(vscmod,'Phasor I-1st')
      |         wn_pll = 'off';
      |         wsw = 'off';
      |         tfilt = 'off';
      |     elseif strcmp(vscmod,'Phasor I-ref')
      |         wn_pll = 'off';
      |         wsw = 'off';
      |         tfilt = 'off';
      |     elseif strcmp(vscmod,'Phasor PQ-1st')
      |         wn_pll = 'off';
      |         wsw = 'off';
      |         tfilt = 'off';
      |     end
      | 
      | fdroop_en = get_param(gcb,'fdroop_en');
      | Vacdroop_en = get_param(gcb,'Vacdroop_en');
      | LVRT_en = get_param(gcb,'LVRT_en');
      | negseq_en = get_param(gcb,'negseq_en');
      | qmode_str = get_param(gcb,'qmode');
      | 
      | 
      | if strcmp(qmode_str,'DC voltage')
      |     DC_en = 'on';
      | else
      |     DC_en = 'off';
      | end
      | 
      | % Set the 'MaskVisibilities' property for each parameters
      |     set_param(gcb,'MaskVisibilities',{'on','on','on','on','on','on','on','on','on',wsw,wn_pll,'on','on','on','on',DC_en,tfilt,'on','on','on','on',fdroop_en,fdroop_en,Vacdroop_en,Vacdroop_en,'on','on','on','on','on','on','on'});
      | 
      | % Make LVRT area visible when it is enabled
      | if strcmp(LVRT_en,'on')
      |   maskObj.getDialogControl('Container_LVRT').Visible = 'on';
      | else
      |     maskObj.getDialogControl('Container_LVRT').Visible = 'off';
      | end
      | 
      | % Note that the value of the bias is not handled here.
      | % See the Initialization tab
      mask DialogControl DescTextVar Prompt: -------------------------------------Three-phase VSC model---------------------------------------
      mask DialogControl Tab1 Prompt: Electrical parameters
      mask DialogControl Tab2 Prompt: Control parameters
      mask DialogControl Tab3 Prompt: Other parameters
      mask DialogControl Container_LVRT Prompt: LVRT
      mask DialogControl Tab4 Prompt: Power flow
      mask Display:
      | choice = get_param(gcb,'vscmod');
      | if strcmp(choice,'Phasor Quasi-EMT')
      |     disp('VSC\n\n')
      |     disp('\n\nPhasor\n\n')
      |     disp('\n\nQuasi-EMT')
      | elseif strcmp(choice,'EMT Average')
      |     disp('VSC\n')
      |     disp('\nEMT AVG')
      | elseif strcmp(choice,'EMT Switching')
      |     disp('VSC\n')
      |     disp('\nEMT SW')
      | elseif strcmp(choice,'Phasor I-1st')
      |     disp('VSC\n\n')
      |     disp('\n\nPhasor\n\n')
      |     disp('\n\nI 1st')
      | elseif strcmp(choice,'Phasor I-ref')
      |     disp('VSC\n\n')
      |     disp('\n\nPhasor\n\n')
      |     disp('\n\nI ref')
      | elseif strcmp(choice,'Phasor PQ-1st')
      |     disp('VSC\n\n')
      |     disp('\n\nPhasor\n\n')
      |     disp('\n\nPQ 1st')
      | end
  A : PMIOPort  Side=Right
  B : PMIOPort  Port=2  Side=Right
  C : PMIOPort  Port=3  Side=Right
  tag scope: Pg11=global, Qg11=global, fg11=global
  wires:
  VSC v2/1(m) -> Bus Selector/1
  Bus Selector/2 -> [Qg11]  "<Qabc>"
  Bus Selector/1 -> [Pg11]  "<Pabc>"
  Bus Selector/3 -> [fg11]  "<f>"
  Constant/1 -> VSC v2/1(Pset)
  Constant1/1 -> VSC v2/2(Qset)
  connections:
  VSC v2/LConn2 -- B/RConn1
  VSC v2/LConn1 -- A/RConn1
  VSC v2/LConn3 -- C/RConn1
